simulink model "diskret_modell_1"  (Simulink 7.8)
settings: Solver=ode45  StartTime=0.0  StopTime=0.1  RelTol=1e-3
libraries: dspsigops x1
settings Model: Creator=josef  LastModifiedBy=josef

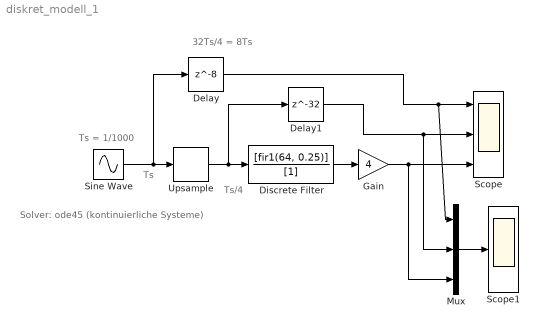
== system diskret_modell_1 ==
  note: Ts = 1/1000
  note: Ts/4
  note: Solver: ode45
      |  (kontinuierliche Systeme)
  note: 32Ts/4 = 8Ts
  note: Ts
  Delay : Delay  DelayLength=8
  Delay1 : Delay  DelayLength=32
  Discrete Filter : DiscreteFilter  Numerator=[fir1(64, 0.25)]  Denominator=[1]
  Gain : Gain  Gain=4
  Mux : Mux  Inputs=3
  Scope : Scope  NumInputPorts=3
      settings: TimeRange=0.03999999999999999  YMin=-5~-5~-2  YMax=5~5~2
  Scope1 : Scope
      settings: TimeRange=0.03999999999999999
  Sine Wave : Sin  Frequency=2*pi*200  SampleTime=1/1000
  Upsample : dspsigops/Upsample  N=4  phase=0  RateOptions=Allow multirate processing  ic=0  mode=Unused parameter value
  wires:
  Sine Wave/1 -> Upsample/1, Delay/1
  Upsample/1 -> Discrete Filter/1, Delay1/1
  Discrete Filter/1 -> Gain/1
  Gain/1 -> Scope/3, Mux/3
  Delay1/1 -> Scope/2, Mux/2
  Delay/1 -> Scope/1, Mux/1
  Mux/1 -> Scope1/1
